simulink model "FJR_Baseline"  (R2025b)
settings: Solver=ode45  StartTime=0.0  StopTime=10.0  MaxStep=0.001  RelTol=1e-3
values from neighbouring files (symbols this model uses):
  B_j = 0.5    [FJR_plant_params.m]
  B_l = 0.2    [FJR_plant_params.m]
  B_m = 0.2    [FJR_plant_params.m]
  J_l = 1.0    (= 1)    [FJR_plant_params.m]
  J_m = 0.5    [FJR_plant_params.m]
  K = 10.0    (= 10)    [FJR_plant_params.m]
  Ks = 0.7    [FJR_ctrl_classical.m]    (also in FJR_ctrl_sat.m = 0.9; FJR_ctrl_tanh.m = 0.9; FJR_ctrl_vbsmc.m)
  lambda = 3.5    [FJR_ctrl_classical.m]    (also in FJR_ctrl_sat.m = 3; FJR_ctrl_tanh.m = 3; FJR_ctrl_vbsmc.m = 3)
settings Model: Creator=Shreya  LastModifiedBy=Shreya

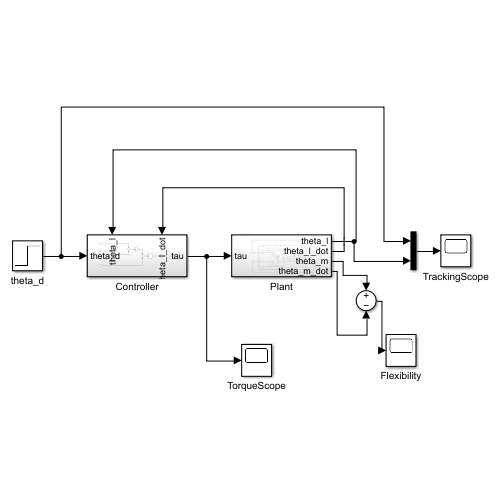
[thumbnail: Simulink's stored preview of the top-level diagram]
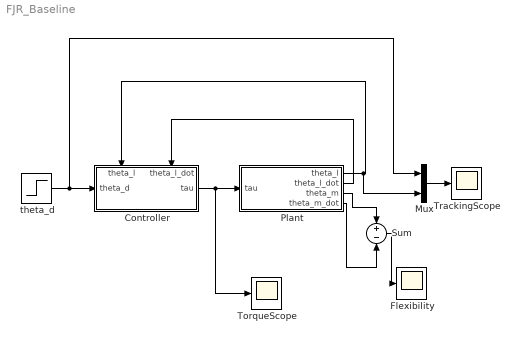
== system FJR_Baseline ==
  Controller : Subsystem
      settings: PortSchema="{\"entries\":[{\"content\":{\"sides\":[{\"content\":{\"connectorIds\":[\"In1\"]},\"type\":\"ConnectorPlacement.EquallySpacedRectSide\",\"uuid\":\"a9f27d26-72ba-436d-acce-42d3067e67ca\"},{\"content\":{\"connectorIds\":[\"Out1\"],\"side\":\"RIGHT\"},\"type\":\"ConnectorPlacement.EquallySpacedRectSide\",\"uuid\":\"30cedea4-f33e-40bd-a8c5-bb3e70fa47eb\"},{\"content\":{\"connectorIds\":[\"In2\",\"In3\"],\"side\":\"TOP\"},\"type\":\"ConnectorPlacement.EquallySpacedRectSide\",\"uuid\":\"113d62d2-1248-4e63-9237-9801a09bb6b1\"},{\"content\":{\"side\":\"BOTTOM\"},\"type\":\"ConnectorPlacement.EquallySpacedRectSide\",\"uuid\":\"8f01fa0c-68f7-455d-b313-c079313a1fd6\"}]},\"type\":\"ConnectorPlacement.EquallySpacedConnector\",\"uuid\":\"694d89f6-7997-4a7b-af3b-bac990d97b9a\"}],\"packageUris\":[\"http://schema.mathworks.com/mf0/Connector/R2020b\"],\"version\":\"1.0\"}"
  Flexibility : Scope
      settings: ActiveDisplayYMinimum=-0.045342743465751331  ActiveDisplayYMaximum=0.28711517932171354  DataLoggingVariableName=ScopeData2
  Mux : Mux  Inputs=2
  Plant : Subsystem
  Sum : Sum  Inputs=+-
  TorqueScope : Scope
      settings: ActiveDisplayYMinimum=-1.0080012077294684  ActiveDisplayYMaximum=0.9213737922705314
  TrackingScope : Scope
      settings: ActiveDisplayYMinimum=-0.030707912054213984  ActiveDisplayYMaximum=0.2763712084879259
  theta_d : Step  After=0.2  SampleTime=0
  wires:
  theta_d/1 -> Controller/1(theta_d), Mux/1
  Controller/1(tau) -> TorqueScope/1, Plant/1(tau)
  Plant/1(theta_l) -> Mux/2, Controller/2(theta_l)
  Plant/2(theta_l_dot) -> Controller/3(theta_l_dot)
  Mux/1 -> TrackingScope/1
  Plant/3(theta_m) -> Sum/1
  Plant/4(theta_m_dot) -> Sum/2
  Sum/1 -> Flexibility/1

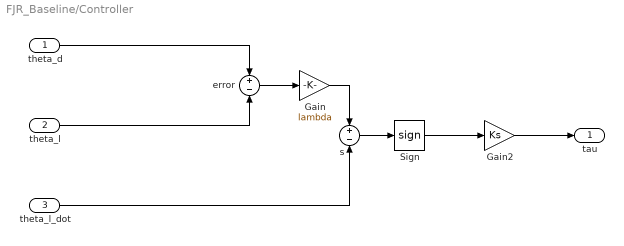
== system FJR_Baseline/Controller ==
  theta_d : Inport
  theta_l : Inport  Port=2
  theta_l_dot : Inport  Port=3
  Gain : Gain  Gain=lambda
  Gain2 : Gain  Gain=Ks
  Sign : Signum
  error : Sum  Inputs=+-
  s : Sum  Inputs=+-
  tau : Outport
  wires:
  theta_d/1 -> error/1
  theta_l/1 -> error/2
  error/1 -> Gain/1
  theta_l_dot/1 -> s/2
  Gain/1 -> s/1
  s/1 -> Sign/1
  Gain2/1 -> tau/1
  Sign/1 -> Gain2/1

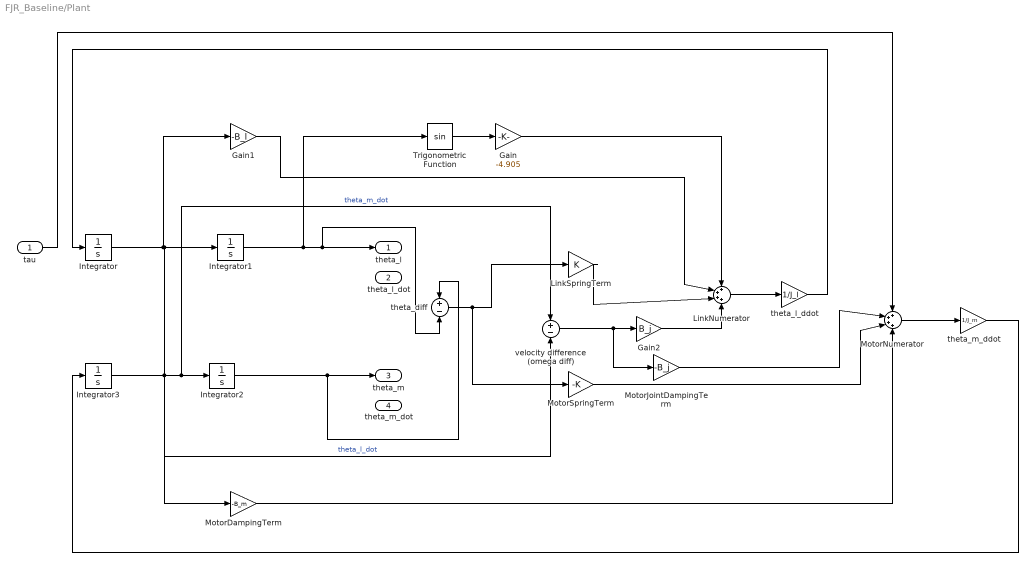
== system FJR_Baseline/Plant ==
  tau : Inport
  Gain : Gain  Gain=-4.905
  Gain1 : Gain  Gain=-B_l
  Gain2 : Gain  Gain=B_j
  Integrator{,1..3} (4 alike) : Integrator
  LinkNumerator : Sum  Inputs=++++
  LinkSpringTerm : Gain  Gain=K
  MotorDampingTerm : Gain  Gain=-B_m
  MotorJointDampingTerm : Gain  Gain=-B_j
  MotorNumerator : Sum  Inputs=++++
  MotorSpringTerm : Gain  Gain=-K
  Trigonometric Function : Trigonometry
  theta_diff : Sum  Inputs=+-
  theta_l_ddot : Gain  Gain=1/J_l
  theta_m_ddot : Gain  Gain=1/J_m
  velocity difference (omega diff) : Sum  Inputs=+-
  theta_l : Outport
  theta_l_dot : Outport  Port=2
  theta_m : Outport  Port=3
  theta_m_dot : Outport  Port=4
  wires:
  Integrator/1 -> velocity difference (omega diff)/2, Integrator1/1, Gain1/1  "theta_l_dot"
  Integrator3/1 -> MotorDampingTerm/1, Integrator2/1, velocity difference (omega diff)/1  "theta_m_dot"
  Integrator1/1 -> Trigonometric Function/1, theta_l/1, theta_diff/2
  Integrator2/1 -> theta_m/1, theta_diff/1
  Trigonometric Function/1 -> Gain/1
  theta_diff/1 -> MotorSpringTerm/1, LinkSpringTerm/1
  velocity difference (omega diff)/1 -> MotorJointDampingTerm/1, Gain2/1
  Gain/1 -> LinkNumerator/1
  Gain1/1 -> LinkNumerator/2
  LinkSpringTerm/1 -> LinkNumerator/3
  Gain2/1 -> LinkNumerator/4
  LinkNumerator/1 -> theta_l_ddot/1
  theta_l_ddot/1 -> Integrator/1
  tau/1 -> MotorNumerator/1
  MotorDampingTerm/1 -> MotorNumerator/4
  MotorSpringTerm/1 -> MotorNumerator/3
  MotorJointDampingTerm/1 -> MotorNumerator/2
  MotorNumerator/1 -> theta_m_ddot/1
  theta_m_ddot/1 -> Integrator3/1
